simulink model "battery_model_test"  (R2019b)
settings: Solver=VariableStepAuto  StartTime=0.0  StopTime=10.0  RelTol=1e-3
undefined symbols (not defined in the file or in its folder): Acid, Lead
libraries: powerlib x5, electricdrivelib x2
settings Model: Creator=root  LastModifiedBy=root

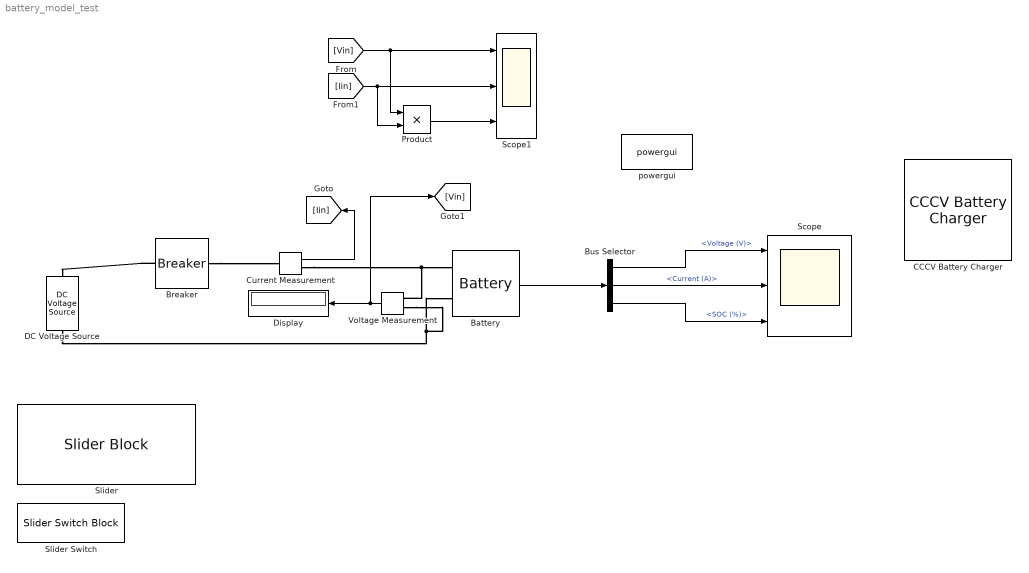
== system battery_model_test ==
  Battery : electricdrivelib/Extra Sources/Battery  BatType=Lead-Acid  ShowTempParam=off  ThermalPreset=no  ShowAgeParam=off  NomV=12  NomQ=40  SOC=90  Batt_Tr=10  PresetModel=on  MaxQ=41.6667  MinV=9  FullV=13.0658  Dis_rate=8  R=0.003  Normal_OP=12.4111  expZone="[12.2171     0.133333]"  current=[6.5 13 32.5]  Units=Time  Tci=20  NomT=20  T2=-30  MaxQ2=4.8  FullV2=7.1  Normal_OP2=5.655  expZone2="[6.58           1]"  Rca=0.6  ti=2000  Dp=0  Neq0=0  Tsim=1e6  Ta1=25  Qeol=5.4*0.9  Reol=0.013333*1.2  Char_age=[2.3478, 3]  Dis_age=[2.3478, 10]  N1=1500  N2=10500  N3=1000  N4=1400  Ta2=45  N5=950
      settings: SourceProductName=Simscape Electrical
  Breaker : powerlib/Elements/Breaker  InitialState=0  SwitchingTimes=[5]  External=off  BreakerResistance=0.001  SnubberResistance=1e6  SnubberCapacitance=inf  Measurements=None  MoreParameters=on  NoBreakLoop=off
      settings: SourceProductName=Simscape Electrical
  Bus Selector : BusSelector  OutputSignals=Voltage (V),Current (A),SOC (%)
  CCCV Battery Charger : electricdrivelib/Extra Sources/CCCV Battery Charger  Preset=Custom specifications  P_nom=1500  s_type=DC  n_connect=off  eff_volt=15  in_freq=60  in_I_ripple=1  in_I_freq=1000  EFF_en=on  EFF_val=[0.627 0.803 0.855 0.871 0.872 0.864]  EFF_fu=[0.063 0.177 0.293 0.483 0.674 0.914]  THD_en=on  I_THD_val=[0.327 0.394 0.394 0.351 0.289 0.265]  I_THD_fu=[0.056 0.136 0.194 0.303 0.555 0.916]  H_DIST_rt=[0.199 1.297 0.328 0.029 0.416 0.200]  H_DIST_fr=[3 5 7 9 11 13]  PF_en=on  PF_val=[0.316 0.532 0.662 0.731 0.780 0.792]  PF_fu=[0.067 0.230 0.445 0.625 0.794 0.919]  Out_mode=Constant Current - Constant Voltage (CCCV)  DynInT=on  I_cst=10  V_cst=138  ABS_en=off  V_abs=142  ABS_end=Time based  ABS_time=3600  ABS_i=40  ripple=0.5  swF=1000  overshoot=1  stable_t=5  VoltComp=on  V_comp=-0.18  nom_temp=20
      settings: SourceProductName=Simscape Electrical  SourceProductBaseCode=PS
  Current Measurement : powerlib/Measurements/Current Measurement  PhasorSimulation=off  OutputType=Complex  PSBequivalent=0
      settings: SourceProductName=Simscape Electrical
  DC Voltage Source : powerlib/Electrical Sources/DC Voltage Source  Amplitude=12.95955882352941  Measurements=None
      settings: SourceProductName=Simscape Electrical
  Display : Display
  Product : Product
  Scope : Scope  NumInputPorts=3
  Scope1 : Scope  NumInputPorts=3
  Slider : SliderBlock
  Slider Switch : SliderSwitchBlock
      settings: Values={{'Off', 'On'}, [0 1]}
  Voltage Measurement : powerlib/Measurements/Voltage Measurement  PhasorSimulation=off  OutputType=Complex  PSBequivalent=0
      settings: SourceProductName=Simscape Electrical
  powergui : powerlib/powergui  Priority=1  SimulationMode=Discrete  SampleTime=10e-6  frequency=60  Iterations=50  frequencyindice=0  Pbase=100e6  ErrMax=1e-4  UnitsV=kV  UnitsW=MW  buscounter=0  FunctionMessages=off  echomessages=off  EnableUseOfTLC=off  CurrentSourceSwitches=off  DisableSnubberDevices=off  DisableRonSwitches=off  DisableVfSwitches=off  DisplayEquations=off  AutomaticDiscreteSolvers=off  SolverType=Tustin/Backward Euler (TBE)  Interpol=off  ExternalGateDelay=off  methode=off  Ts=100  x0status=blocks  SPID=on  SwTol=0  HookPort=off  NonlinearTolerance=1e-4  nMaxIteration=100  ContinueOnMaxIteration=off  RestoreLinks=warning  ResistiveCurrentMeasurement=off  Frange=[0:2:500]  Ylog=off  Xlog=on  ShowGrid=off  save=off  variable=ZData  structure=0  ZoomFFT=off  StartTime=0.0  cycles=1  DisplayStyle=1  fundamental=60  FreqAxis=off  MaxFrequency=1000  frequencyindicesteady=1  RmsSteady=1  display=off
      settings: SourceProductName=Simscape Electrical
  wires:
  Battery/1 -> Bus Selector/1
  Bus Selector/1 -> Scope/1  "<Voltage (V)>"
  Bus Selector/2 -> Scope/2  "<Current (A)>"
  Bus Selector/3 -> Scope/3  "<SOC (%)>"
  Current Measurement/1 -> [Iin]
  Voltage Measurement/1 -> Display/1, [Vin]
  [Vin] -> Product/1, Scope1/1
  [Iin] -> Scope1/2, Product/2
  Product/1 -> Scope1/3
  connections:
  DC Voltage Source/LConn1 -- Voltage Measurement/LConn2 -- Battery/LConn2
  Current Measurement/RConn1 -- Voltage Measurement/LConn1 -- Battery/LConn1
  Breaker/RConn1 -- Current Measurement/LConn1
  Breaker/LConn1 -- DC Voltage Source/RConn1
